simulink model "munge_blk"  (R2019a)
settings: Solver=VariableStepAuto  StartTime=0.0  StopTime=10.0  RelTol=1e-3
libraries: xbsIndex_r4 x4
settings Model: Creator=Ross Donnachie  LastModifiedBy=Ross Donnachie

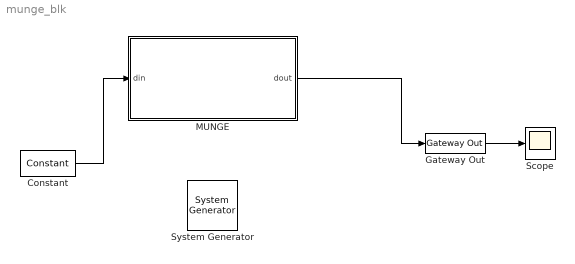
== system munge_blk ==
  " System Generator" : xbsIndex_r4/ System Generator  Tag=genX  xilinxfamily=kintex7  part=xc7k325t  speed=-3  package=fbg676  synthesis_tool=Vivado  clock_wrapper=Clock Enables  directory=./netlist  proj_type=Vivado  Synth_file=Vivado Synthesis Defaults  Impl_file=Vivado Implementation Defaults  testbench=off  simulink_period=1  sysclk_period=10  dcm_input_clock_period=10  incr_netlist=off  trim_vbits=Everywhere in SubSystem  dbl_ovrd=According to Block Masks  core_generation=According to Block Masks  run_coregen=off  deprecated_control=off  eval_field=0  block_type=sysgen
  Constant : xbsIndex_r4/Constant  const=192  gui_display_data_type=Fixed-point  arith_type=Unsigned  n_bits=8  bin_pt=0  preci_type=Single  exp_width=8  frac_width=24  explicit_period=on  period=1  equ=P=C  opselect=C  inp2=PCIN>>17  opr=+  inp1=P  carry=CIN  dbl_ovrd=off  block_type=constant
  Gateway Out : xbsIndex_r4/Gateway Out  inherit_from_input=on  hdl_port=off  rows=1  columns=1  UseAsDAC=off  DACChannel='1'  interface=None  automatic_assignment=on  address_offset=hex2dec('00')  intf_name=''  intf_description=''  timing_constraint=None  locs_specified=off  LOCs={}  io_standard={}  block_type=gatewayout
  "MUNGE " : Subsystem  mask{number_of_divisions=4, division_size_bits=2, packing_order="3,2,0,0"}
      mask prompts: number_of_divisions "Number of equal parts to divide the bits into."; division_size_bits "Number of bits per division."; packing_order "Zero-indexed comma delimited (',') division indices of output. Indices >= zero, no spaces."
      mask init:
      | Simulink.Block.eval([gcb, '/munge']);
      mask DialogControl DescTextVar Prompt: A block that reorders bits.
  Scope : Scope
  wires:
  Constant/1 -> "MUNGE "/1(din)
  "MUNGE "/1(dout) -> Gateway Out/1
  Gateway Out/1 -> Scope/1

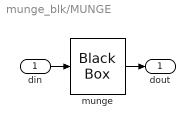
== system munge_blk/MUNGE  ==
  din : Inport
  munge : xbsIndex_r4/Black Box  init_code=munge_config  sim_method=ISE Simulator  verbose=on  block_type=blackbox2
  dout : Outport
  wires:
  munge/1 -> dout/1
  din/1 -> munge/1
